simulink model "general_charger_2_cc_cv_test"  (R2013a)
settings: Solver=ode23  StartTime=0  StopTime=1.5  RelTol=1e-3
PreLoadFcn:
  | Ts =5e-6;
values from neighbouring files (symbols this model uses):
  ac_volt = 169    [charger_init.m]    (also in charger_init_simpl.m)
  acdc_on_time = 0.2    [charger_init.m]    (also in charger_init_simpl.m = 0)
  Cdc = 2e-3    (= 0.002)    [charger_init.m]    (also in charger_init_simpl.m)
  dcAd = dcinvexp*(eye(dcnstates) + (Ts/2)*dcAc)    [charger_init.m]    (also in charger_init_simpl.m)
  dcBd = dcinvexp*dcBc    [charger_init.m]    (also in charger_init_simpl.m)
  dcCd = dcCc*dcinvexp*Ts    [charger_init.m]    (also in charger_init_simpl.m)
  dcDd = dcCc*dcinvexp*dcBc*(Ts/2) + dcDc    [charger_init.m]    (also in charger_init_simpl.m)
  ESLCd = 0.1e-9    (= 1e-10)    [charger_init.m]    (also in charger_init_simpl.m)
  ESRCd = 70e-3    (= 0.07)    [charger_init.m]    (also in charger_init_simpl.m)
  ESRLdcdc = 0.1    [charger_init.m]    (also in charger_init_simpl.m)
  ESRLin = 0.2    [charger_init.m]    (also in charger_init_simpl.m = 0.1)
  Ldcdc = 1.3e-3    (= 0.0013)    [charger_init.m]    (also in charger_init_simpl.m = 0.0014)
  Lin = 1.5e-3    (= 0.0015)    [charger_init.m]    (also in charger_init_simpl.m = 0.001)
  P = 1.92e3    (= 1920)    [charger_init.m]    (also in charger_init_simpl.m)
  Q = 0    [charger_init.m]    (also in charger_init_simpl.m)
  ramp = (dc_volt - Vdcmin)/(acdc_ramp_end_time)    (= 202)    [charger_init.m]    (also in charger_init_simpl.m = (dc_volt - Vdcmin)/(acdc_ramp_end_time))
  Rbatt = 0.20    (= 0.2)    [charger_init.m]    (also in charger_init_simpl.m = 0.1)
  switch_Ts = 5e-5    (= 5e-05)    [charger_init.m]    (also in charger_init_simpl.m)
  sys_Ts = 5e-6    (= 5e-06)    [charger_init.m]    (also in charger_init_simpl.m)
  Vdcmin = ac_volt + 10    (= 179)    [charger_init.m]    (also in charger_init_simpl.m)
  voc = 105    [charger_init.m]    (also in charger_init_simpl.m)
undefined symbols (not defined in the file or in its folder): CESR, cpi
undefined symbols (not defined in the file): active_power_on, Ad, Bd, Cd, dc_volt, dcdc_cc_ref, dcdc_cv_ref, dcdc_iki, dcdc_ikp, dcdc_on, dcdc_vki, dcdc_vkp, Dd, dq_id_ki, dq_id_kp, dq_iq_ki, dq_iq_kp, dq_vdc_ki, dq_vdc_kp, dqQ_ki, dqQ_kp, P_ki, P_kp, pi_iac_ki, pi_iac_kp, pi_vdc_ki, pi_vdc_kp, piQ_ki, piQ_kp, pr_iac_kp, pr_pr_ki, pr_pr_kp, pr_vdc_ki, pr_vdc_kp, reactive_power_on
libraries: simulink_extras x165, powerlib x61, simulink x35, powerlib_meascontrol x11
(part 7 of 7)

== system general_charger_2_cc_cv_test/control_stage/AC//DC Control/PR Controller/PR Controller/PLL/AB->DQ/Vq Discretization Error Correction/RMS4 ==
  ac in : Inport
  Constant : Constant  Value=K1
  Constant1 : Constant  Value=f  SampleTime=-1
  Constant2 : Constant  Value=K2
  Delay : Delay  DelayLength=ceil(SpC)  SampleTime=rms_Ts
  Gain : Gain  Gain=K1  SaturateOnIntegerOverflow=on  OutDataTypeStr=Inherit: Same as input  ParamDataTypeStr=Inherit: Same as input
  Gain1 : Gain  Gain=K2  SaturateOnIntegerOverflow=on  OutDataTypeStr=Inherit: Same as input  ParamDataTypeStr=Inherit: Same as input
  PI3 : Subsystem  mask{ki=1, kp=0, Ts_pi=rms_Ts, int_sat_up=inf, int_sat_low=-inf, pi_sat_up=inf, pi_sat_low=-inf}
      mask prompts: ki "Integral Gain"; kp "Proportional Gain"; Ts_pi "Sample Time"; int_sat_up "Integral Saturation Upper"; int_sat_low "Integral Saturation Lower"; pi_sat_up "PI Controller Saturation Upper"; pi_sat_low "PI Controller Saturation Lower"
      mask Display: disp('PI')
  Product3 : Product  SaturateOnIntegerOverflow=on  InputSameDT=on  OutDataTypeStr=Inherit: Same as first input
  Product4 : Product  SaturateOnIntegerOverflow=on  InputSameDT=on  OutDataTypeStr=Inherit: Same as first input
  Pulse Generator : DiscretePulseGenerator  Period=rms_Ts/sys_Ts  SampleTime=sys_Ts
  Sample and Hold : powerlib_meascontrol/Additional Components/Sample and Hold  ic=0  Ts=sys_Ts
  Saturation : Saturate  UpperLimit=inf  LowerLimit=0
  Scope : Scope  NumInputPorts=2
      settings: YMin=-5~-5  YMax=5~5  SaveName=ScopeData2
  Sqrt : Sqrt  SaturateOnIntegerOverflow=on
  Sum1 : Sum  Inputs=+-  SaturateOnIntegerOverflow=on  InputSameDT=on  OutDataTypeStr=Inherit: Same as first input
  Sum2 : Sum  Inputs=-+  SaturateOnIntegerOverflow=on  InputSameDT=on  OutDataTypeStr=Inherit: Same as first input
  Sum3 : Sum  SaturateOnIntegerOverflow=on  InputSameDT=on  OutDataTypeStr=Inherit: Same as first input
  Unit Delay : UnitDelay  SampleTime=rms_Ts
  rms out : Outport
  wires:
  Sum2/1 -> Product4/1
  Constant1/1 -> Product4/2
  Delay/1 -> Sum2/1
  Product3/1 -> Unit Delay/1, Gain1/1, PI3/1(in)
  PI3/1(out) -> Sum2/2, Delay/1
  Sqrt/1 -> rms out/1
  Gain1/1 -> Sum1/1
  Unit Delay/1 -> Gain/1
  Gain/1 -> Sum1/2
  Product4/1 -> Sum3/1
  Sum3/1 -> Saturation/1
  Sum1/1 -> Sum3/2  "Correction"
  Saturation/1 -> Sqrt/1
  Pulse Generator/1 -> Sample and Hold/2
  Sample and Hold/1 -> Product3/1, Product3/2
  ac in/1 -> Sample and Hold/1
  Constant2/1 -> Scope/2
  Constant/1 -> Scope/1

== system general_charger_2_cc_cv_test/control_stage/AC//DC Control/DQ Controller/AB-DQ Transform/PLL/AB->DQ/Vd Discretization Error Correction/RMS4/PI3 ==
  in : Inport
  Add1 : Sum
  Add2 : Sum
  Ki : Gain  Gain=ki
  Kp : Gain  Gain=kp
  Tappe : simulink/Discrete/Tapped Delay  vinit=0.0  samptime=Ts_pi  NumDelays=1  DelayOrder=Oldest  includeCurrent=off
  Ts : Gain  Gain=Ts_pi
  integral saturation : Saturate  UpperLimit=int_sat_up  LowerLimit=int_sat_low  SampleTime=Ts_pi
  pi controller saturation : Saturate  UpperLimit=pi_sat_up  LowerLimit=pi_sat_low  SampleTime=Ts_pi
  out : Outport
  wires:
  Ts/1 -> Ki/1
  in/1 -> Kp/1, Ts/1  "vdc_error"
  Add1/1 -> integral saturation/1  "vdc_int_pi"
  Kp/1 -> Add2/2  "vdc_kp_pi"
  pi controller saturation/1 -> out/1
  Tappe/1 -> Add1/1
  Add2/1 -> pi controller saturation/1  "vdc_pi"
  Ki/1 -> Add1/2
  integral saturation/1 -> Add2/1, Tappe/1

== system general_charger_2_cc_cv_test/control_stage/AC//DC Control/DQ Controller/AB-DQ Transform/PLL/AB->DQ/Vq Discretization Error Correction/RMS4/PI3 ==
  in : Inport
  Add1 : Sum
  Add2 : Sum
  Ki : Gain  Gain=ki
  Kp : Gain  Gain=kp
  Tappe : simulink/Discrete/Tapped Delay  vinit=0.0  samptime=Ts_pi  NumDelays=1  DelayOrder=Oldest  includeCurrent=off
  Ts : Gain  Gain=Ts_pi
  integral saturation : Saturate  UpperLimit=int_sat_up  LowerLimit=int_sat_low  SampleTime=Ts_pi
  pi controller saturation : Saturate  UpperLimit=pi_sat_up  LowerLimit=pi_sat_low  SampleTime=Ts_pi
  out : Outport
  wires:
  Ts/1 -> Ki/1
  in/1 -> Kp/1, Ts/1  "vdc_error"
  Add1/1 -> integral saturation/1  "vdc_int_pi"
  Kp/1 -> Add2/2  "vdc_kp_pi"
  pi controller saturation/1 -> out/1
  Tappe/1 -> Add1/1
  Add2/1 -> pi controller saturation/1  "vdc_pi"
  Ki/1 -> Add1/2
  integral saturation/1 -> Add2/1, Tappe/1

== system general_charger_2_cc_cv_test/control_stage/AC//DC Control/PR Controller/PR Controller/PLL/AB->DQ/Vd Discretization Error Correction/RMS4/PI3 ==
  in : Inport
  Add1 : Sum
  Add2 : Sum
  Ki : Gain  Gain=ki
  Kp : Gain  Gain=kp
  Tappe : simulink/Discrete/Tapped Delay  vinit=0.0  samptime=Ts_pi  NumDelays=1  DelayOrder=Oldest  includeCurrent=off
  Ts : Gain  Gain=Ts_pi
  integral saturation : Saturate  UpperLimit=int_sat_up  LowerLimit=int_sat_low  SampleTime=Ts_pi
  pi controller saturation : Saturate  UpperLimit=pi_sat_up  LowerLimit=pi_sat_low  SampleTime=Ts_pi
  out : Outport
  wires:
  Ts/1 -> Ki/1
  in/1 -> Kp/1, Ts/1  "vdc_error"
  Add1/1 -> integral saturation/1  "vdc_int_pi"
  Kp/1 -> Add2/2  "vdc_kp_pi"
  pi controller saturation/1 -> out/1
  Tappe/1 -> Add1/1
  Add2/1 -> pi controller saturation/1  "vdc_pi"
  Ki/1 -> Add1/2
  integral saturation/1 -> Add2/1, Tappe/1

== system general_charger_2_cc_cv_test/control_stage/AC//DC Control/PR Controller/PR Controller/PLL/AB->DQ/Vq Discretization Error Correction/RMS4/PI3 ==
  in : Inport
  Add1 : Sum
  Add2 : Sum
  Ki : Gain  Gain=ki
  Kp : Gain  Gain=kp
  Tappe : simulink/Discrete/Tapped Delay  vinit=0.0  samptime=Ts_pi  NumDelays=1  DelayOrder=Oldest  includeCurrent=off
  Ts : Gain  Gain=Ts_pi
  integral saturation : Saturate  UpperLimit=int_sat_up  LowerLimit=int_sat_low  SampleTime=Ts_pi
  pi controller saturation : Saturate  UpperLimit=pi_sat_up  LowerLimit=pi_sat_low  SampleTime=Ts_pi
  out : Outport
  wires:
  Ts/1 -> Ki/1
  in/1 -> Kp/1, Ts/1  "vdc_error"
  Add1/1 -> integral saturation/1  "vdc_int_pi"
  Kp/1 -> Add2/2  "vdc_kp_pi"
  pi controller saturation/1 -> out/1
  Tappe/1 -> Add1/1
  Add2/1 -> pi controller saturation/1  "vdc_pi"
  Ki/1 -> Add1/2
  integral saturation/1 -> Add2/1, Tappe/1
